simulink model "Convert_kg_to_pounds"  (R2022b)
settings: Solver=VariableStepAuto  StartTime=0.0  StopTime=10.0  RelTol=1e-3
settings Model: Creator=Dell  LastModifiedBy=Dell

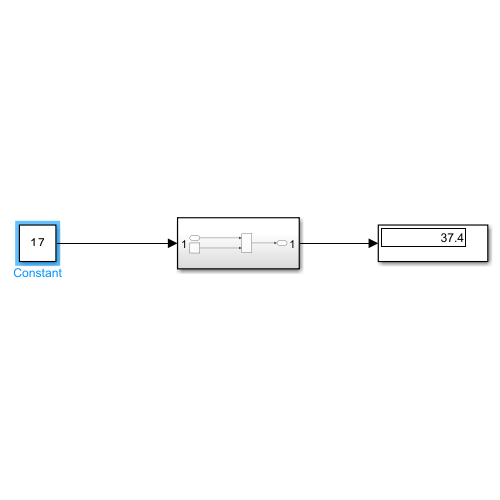
[thumbnail: Simulink's stored preview of the top-level diagram]
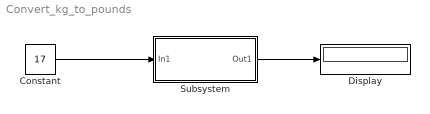
== system Convert_kg_to_pounds ==
  Constant : Constant  Value=17
  Display : Display
  Subsystem : Subsystem
  wires:
  Constant/1 -> Subsystem/1(In1)
  Subsystem/1(Out1) -> Display/1

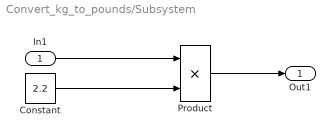
== system Convert_kg_to_pounds/Subsystem ==
  In1 : Inport
  Constant : Constant  Value=2.2
  Product : Product
  Out1 : Outport
  wires:
  In1/1 -> Product/1
  Product/1 -> Out1/1
  Constant/1 -> Product/2
